simulink model "comparacao"  (R2018a)
settings: Solver=ode45  StartTime=0.0  StopTime=1  RelTol=1e-5  EnableMultiTasking=on
undefined symbols (not defined in the file): KIm, Km, KPm, Pm, Ts
libraries: simulink x10
settings Model: Creator=dwbertol  LastModifiedBy=bruno
settings DataIOCC: LimitDataPoints=on  SaveFormat=Array  SignalLoggingSaveFormat=ModelDataLogs
settings OptimizationCC: ExpressionDepthLimit=2147483647  LifeSpan=inf
settings DebuggingCC: UnderspecifiedInitializationDetection=Classic  MergeDetectMultiDrivingBlocksExec=none  SolverPrmCheckMsg=warning  FcnCallInpInsideContextMsg=warning  StateNameClashWarn=warning  SFUnexpectedBacktrackingDiag=warning  SFNoUnconditionalDefaultTransitionDiag=warning  SFExecutionAtInitializationDiag=none
settings HardwareCC: ProdBitPerPointer=32  ProdBitPerSizeT=32  ProdBitPerPtrDiffT=32  ProdLargestAtomicFloat=None  ProdIntDivRoundTo=Undefined  ProdEndianess=Unspecified  ProdWordSize=32  ProdHWDeviceType=32-bit Generic
settings ModelReferenceCC: PropagateSignalLabelsOutOfModel=off
settings CodeAppCC: StateflowObjectComments=on
settings GRTTargetCC: TargetLangStandard=C89/C90 (ANSI)  GeneratePreprocessorConditionals=Disable all  CombineOutputUpdateFcns=off  GRTInterface=on
settings ConfigComp: CovMetricSettings=dw  CovHtmlReporting=on  CovSaveCumulativeToWorkspaceVar=on  CovSaveSingleToWorkspaceVar=on  CovExternalEMLEnable=off

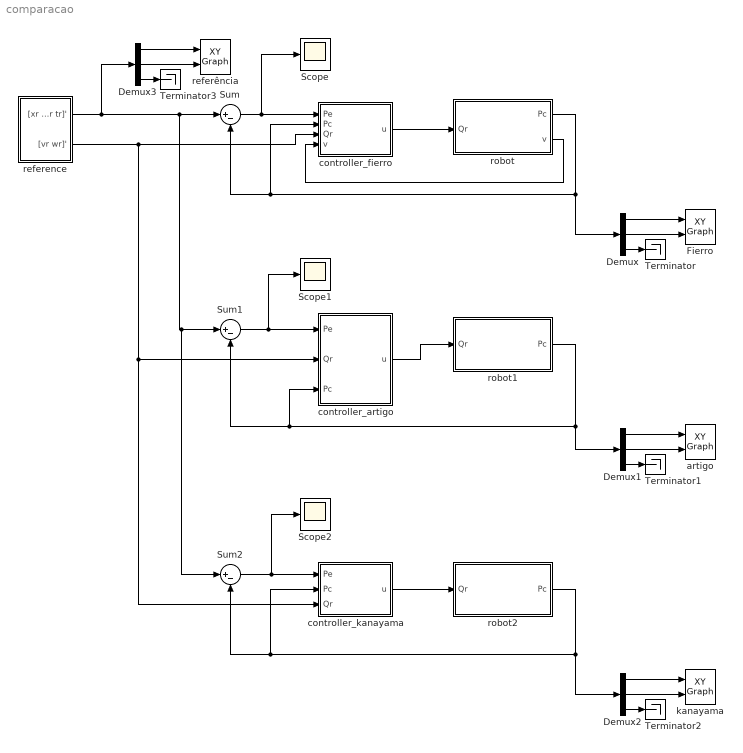
== system comparacao ==
  Demux{,1..3} (4 alike) : Demux  Outputs=3
  Fierro : simulink/Sinks/XY Graph  xmin=-0.1  xmax=1.1  ymin=-0.1  ymax=0.1  st=Ts
  Scope : Scope
  Scope1 : Scope
  Scope2 : Scope
  Sum : Sum  Inputs=|+-  AccumDataTypeStr=double
  Sum1 : Sum  Inputs=|+-  AccumDataTypeStr=double
  Sum2 : Sum  Inputs=|+-  AccumDataTypeStr=double
  Terminator{,1..3} (4 alike) : Terminator
  artigo : simulink/Sinks/XY Graph  xmin=-0.1  xmax=1.1  ymin=-0.1  ymax=0.1  st=Ts
  controller_artigo : Subsystem  mask{k1=60, k2=1000}
  controller_fierro : Subsystem  mask{kx=80, ky=2000, kt=160, k4=400}
  controller_kanayama : Subsystem  mask{kx=80, ky=2000, kt=160}
  kanayama : simulink/Sinks/XY Graph  xmin=-0.1  xmax=1.1  ymin=-0.1  ymax=0.1  st=Ts
  reference : Subsystem  mask{vr=1, wr=0, ini=[0 0.04 0], Ts=Ts}
  referência : simulink/Sinks/XY Graph  xmin=-0.1  xmax=1.1  ymin=-0.1  ymax=0.1  st=Ts
  robot : Subsystem  mask{ini=[0 0 0]'}
  robot1 : Subsystem  mask{ini=[0 0 0]'}
  robot2 : Subsystem  mask{ini=[0 0 0]'}
  wires:
  controller_fierro/1(u) -> robot/1(Qr)
  Demux/3 -> Terminator/1
  Demux/2 -> Fierro/2
  Demux/1 -> Fierro/1
  reference/1("[xr yr tr]' ") -> Demux3/1, Sum2/1, Sum1/1, Sum/1
  Sum/1 -> Scope/1, controller_fierro/1(Pe)
  reference/2("[vr wr]'") -> controller_artigo/2(Qr), controller_kanayama/3(Qr), controller_fierro/3(Qr)
  robot/1(Pc) -> Demux/1, Sum/2, controller_fierro/2(Pc)
  robot/2(v) -> controller_fierro/4(v)
  Demux1/1 -> artigo/1
  Sum1/1 -> Scope1/1, controller_artigo/1(Pe)
  robot1/1(Pc) -> Demux1/1, controller_artigo/3(Pc), Sum1/2
  Demux1/3 -> Terminator1/1
  controller_artigo/1(u) -> robot1/1(Qr)
  Demux1/2 -> artigo/2
  Demux2/1 -> kanayama/1
  Sum2/1 -> Scope2/1, controller_kanayama/1(Pe)
  Demux2/2 -> kanayama/2
  robot2/1(Pc) -> Demux2/1, Sum2/2, controller_kanayama/2(Pc)
  controller_kanayama/1(u) -> robot2/1(Qr)
  Demux2/3 -> Terminator2/1
  Demux3/1 -> referência/1
  Demux3/3 -> Terminator3/1
  Demux3/2 -> referência/2

== system comparacao/controller_artigo ==
  Pe : Inport
  Qr : Inport  Port=2
  Pc : Inport  Port=3
  Constant : Constant  Value=k1
  Constant1 : Constant  Value=k2
  controller : MATLAB Function  TreatAsAtomicUnit=on
  u : Outport
  wires:
  Qr/1 -> controller/2(Qr)
  Pe/1 -> controller/1(Pe)
  controller/1(u) -> u/1
  Constant/1 -> controller/4(k1)
  Constant1/1 -> controller/5(k2)
  Pc/1 -> controller/3(Pc)

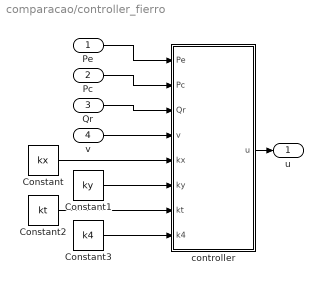
== system comparacao/controller_fierro ==
  Pe : Inport
  Pc : Inport  Port=2
  Qr : Inport  Port=3
  v : Inport  Port=4
  Constant : Constant  Value=kx
  Constant1 : Constant  Value=ky
  Constant2 : Constant  Value=kt
  Constant3 : Constant  Value=k4
  controller : MATLAB Function  TreatAsAtomicUnit=on
  u : Outport
  wires:
  controller/1(u) -> u/1
  Pe/1 -> controller/1(Pe)
  Pc/1 -> controller/2(Pc)
  Qr/1 -> controller/3(Qr)
  v/1 -> controller/4(v)
  Constant/1 -> controller/5(kx)
  Constant1/1 -> controller/6(ky)
  Constant2/1 -> controller/7(kt)
  Constant3/1 -> controller/8(k4)

== system comparacao/controller_kanayama ==
  Pe : Inport
  Pc : Inport  Port=2
  Qr : Inport  Port=3
  controller : MATLAB Function  TreatAsAtomicUnit=on
  u : Outport
  wires:
  Qr/1 -> controller/3(Qr)
  Pc/1 -> controller/2(Pc)
  Pe/1 -> controller/1(Pe)
  controller/1(u) -> u/1

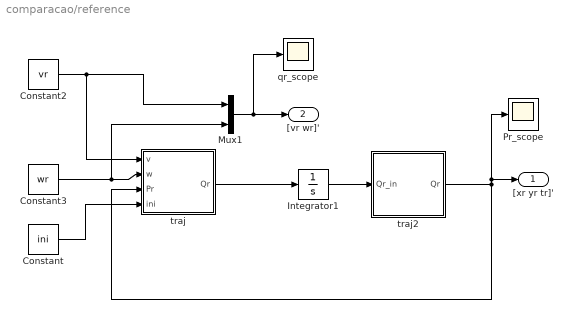
== system comparacao/reference ==
  Constant : Constant  Value=ini
  Constant2 : Constant  Value=vr  VectorParams1D=off
  Constant3 : Constant  Value=wr  VectorParams1D=off
  Integrator1 : Integrator  InitialCondition=ini
  Mux1 : Mux  Inputs=2
  Pr_scope : Scope
  qr_scope : Scope
  traj : MATLAB Function  TreatAsAtomicUnit=on
  traj2 : MATLAB Function  TreatAsAtomicUnit=on
  "[xr yr tr]' " : Outport
  "[vr wr]'" : Outport  Port=2
  wires:
  Integrator1/1 -> traj2/1(Qr_in)
  Constant3/1 -> Mux1/2, traj/2(w)
  Constant2/1 -> traj/1(v), Mux1/1
  Mux1/1 -> "[vr wr]'"/1, qr_scope/1
  traj/1(Qr) -> Integrator1/1
  Constant/1 -> traj/4(ini)
  traj2/1(Qr) -> Pr_scope/1, "[xr yr tr]' "/1, traj/3(Pr)

== system comparacao/robot ==
  Qr : Inport
  Controle velocidades : Subsystem
  Demux2 : Demux  Outputs=[2 1]
  Integrator1 : Integrator  InitialCondition=ini
  J : MATLAB Function  TreatAsAtomicUnit=on
  Terminator : Terminator
  Pc : Outport
  v : Outport  Port=2
  wires:
  J/1(P_ponto) -> Integrator1/1
  Integrator1/1 -> Demux2/1, Pc/1
  Demux2/1 -> Terminator/1
  Qr/1 -> Controle velocidades/1(Qr)
  Controle velocidades/1(Qc) -> v/1, J/1(Qc)
  Demux2/2 -> J/2(teta)

== system comparacao/robot1 ==
  Qr : Inport
  Controle velocidades : Subsystem
  Demux2 : Demux  Outputs=[2 1]
  Integrator1 : Integrator  InitialCondition=ini
  J : MATLAB Function  TreatAsAtomicUnit=on
  Terminator : Terminator
  Pc : Outport
  wires:
  J/1(P_ponto) -> Integrator1/1
  Integrator1/1 -> Demux2/1, Pc/1
  Demux2/1 -> Terminator/1
  Qr/1 -> Controle velocidades/1(Qr)
  Controle velocidades/1(Qc) -> J/1(Qc)
  Demux2/2 -> J/2(teta)

== system comparacao/robot2 ==
  Qr : Inport
  Controle velocidades : Subsystem
  Demux2 : Demux  Outputs=[2 1]
  Integrator1 : Integrator  InitialCondition=ini
  J : MATLAB Function  TreatAsAtomicUnit=on
  Terminator : Terminator
  vel : Scope
  Pc : Outport
  wires:
  J/1(P_ponto) -> vel/1, Integrator1/1
  Integrator1/1 -> Demux2/1, Pc/1
  Demux2/1 -> Terminator/1
  Qr/1 -> Controle velocidades/1(Qr)
  Controle velocidades/1(Qc) -> J/1(Qc)
  Demux2/2 -> J/2(teta)

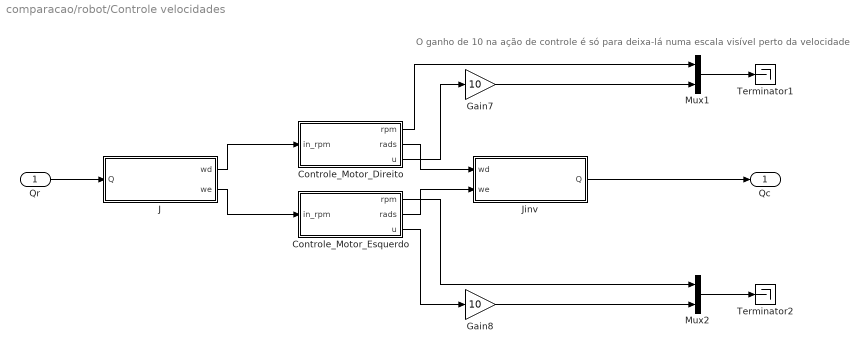
== system comparacao/robot/Controle velocidades ==
  note: O ganho de 10 na ação de controle é só para deixa-lá numa escala visível perto da velocidade
  Qr : Inport
  Controle_Motor_Direito : Subsystem
  Controle_Motor_Esquerdo : Subsystem
  Gain7 : Gain  Gain=10
  Gain8 : Gain  Gain=10
  J : MATLAB Function  TreatAsAtomicUnit=on
  Jinv : MATLAB Function  TreatAsAtomicUnit=on
  Mux1 : Mux  Inputs=2
  Mux2 : Mux  Inputs=2
  Terminator1 : Terminator
  Terminator2 : Terminator
  Qc : Outport
  wires:
  Gain7/1 -> Mux1/2
  Mux2/1 -> Terminator2/1
  Mux1/1 -> Terminator1/1
  Gain8/1 -> Mux2/2
  Controle_Motor_Direito/3(u) -> Gain7/1
  Controle_Motor_Direito/1(rpm) -> Mux1/1
  Controle_Motor_Esquerdo/3(u) -> Gain8/1
  Controle_Motor_Esquerdo/1(rpm) -> Mux2/1
  Qr/1 -> J/1(Q)
  J/1(wd) -> Controle_Motor_Direito/1(in_rpm)
  J/2(we) -> Controle_Motor_Esquerdo/1(in_rpm)
  Controle_Motor_Direito/2(rads) -> Jinv/1(wd)
  Controle_Motor_Esquerdo/2(rads) -> Jinv/2(we)
  Jinv/1(Q) -> Qc/1

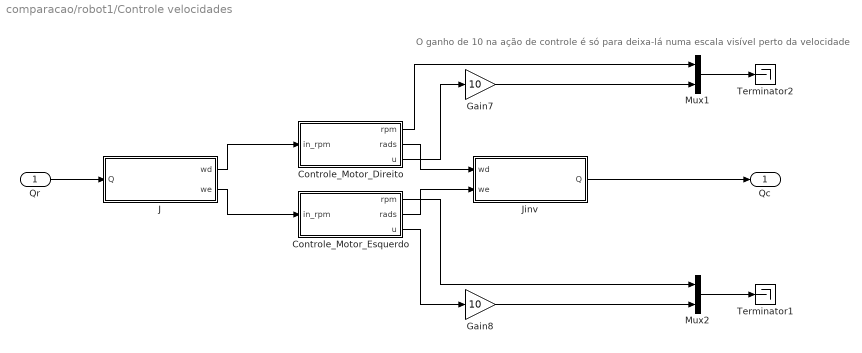
== system comparacao/robot1/Controle velocidades ==
  note: O ganho de 10 na ação de controle é só para deixa-lá numa escala visível perto da velocidade
  Qr : Inport
  Controle_Motor_Direito : Subsystem
  Controle_Motor_Esquerdo : Subsystem
  Gain7 : Gain  Gain=10
  Gain8 : Gain  Gain=10
  J : MATLAB Function  TreatAsAtomicUnit=on
  Jinv : MATLAB Function  TreatAsAtomicUnit=on
  Mux1 : Mux  Inputs=2
  Mux2 : Mux  Inputs=2
  Terminator1 : Terminator
  Terminator2 : Terminator
  Qc : Outport
  wires:
  Gain7/1 -> Mux1/2
  Mux2/1 -> Terminator1/1
  Mux1/1 -> Terminator2/1
  Gain8/1 -> Mux2/2
  Controle_Motor_Direito/3(u) -> Gain7/1
  Controle_Motor_Direito/1(rpm) -> Mux1/1
  Controle_Motor_Esquerdo/3(u) -> Gain8/1
  Controle_Motor_Esquerdo/1(rpm) -> Mux2/1
  Qr/1 -> J/1(Q)
  J/1(wd) -> Controle_Motor_Direito/1(in_rpm)
  J/2(we) -> Controle_Motor_Esquerdo/1(in_rpm)
  Controle_Motor_Direito/2(rads) -> Jinv/1(wd)
  Controle_Motor_Esquerdo/2(rads) -> Jinv/2(we)
  Jinv/1(Q) -> Qc/1

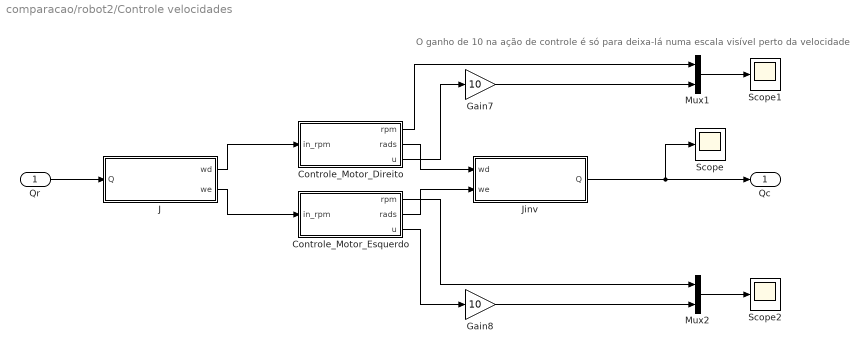
== system comparacao/robot2/Controle velocidades ==
  note: O ganho de 10 na ação de controle é só para deixa-lá numa escala visível perto da velocidade
  Qr : Inport
  Controle_Motor_Direito : Subsystem
  Controle_Motor_Esquerdo : Subsystem
  Gain7 : Gain  Gain=10
  Gain8 : Gain  Gain=10
  J : MATLAB Function  TreatAsAtomicUnit=on
  Jinv : MATLAB Function  TreatAsAtomicUnit=on
  Mux1 : Mux  Inputs=2
  Mux2 : Mux  Inputs=2
  Scope : Scope
  Scope1 : Scope
  Scope2 : Scope
  Qc : Outport
  wires:
  Gain7/1 -> Mux1/2
  Mux2/1 -> Scope2/1
  Mux1/1 -> Scope1/1
  Gain8/1 -> Mux2/2
  Controle_Motor_Direito/3(u) -> Gain7/1
  Controle_Motor_Direito/1(rpm) -> Mux1/1
  Controle_Motor_Esquerdo/3(u) -> Gain8/1
  Controle_Motor_Esquerdo/1(rpm) -> Mux2/1
  Qr/1 -> J/1(Q)
  J/1(wd) -> Controle_Motor_Direito/1(in_rpm)
  J/2(we) -> Controle_Motor_Esquerdo/1(in_rpm)
  Controle_Motor_Direito/2(rads) -> Jinv/1(wd)
  Controle_Motor_Esquerdo/2(rads) -> Jinv/2(we)
  Jinv/1(Q) -> Scope/1, Qc/1

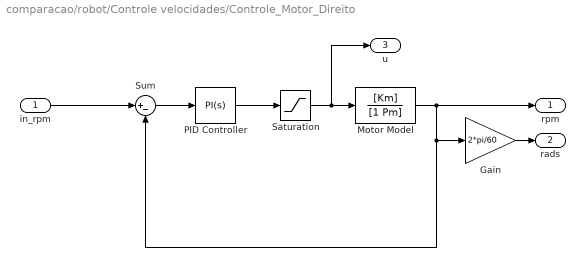
== system comparacao/robot/Controle velocidades/Controle_Motor_Direito ==
  in_rpm : Inport
  Gain : Gain  Gain=2*pi/60
  Motor Model : TransferFcn  Numerator=[Km]  Denominator=[1 Pm]
  PID Controller : simulink/Continuous/PID Controller  Controller=PI  TimeDomain=Continuous-time  SampleTime=-1  IntegratorMethod=Forward Euler  FilterMethod=Forward Euler  Form=Parallel  UseFilter=on  ControllerParametersSource=internal  P=KPm  I=KIm  D=0  N=0  InitialConditionSource=internal  InitialConditionForIntegrator=0  InitialConditionForFilter=0  ExternalReset=none  LimitOutput=off  UpperSaturationLimit=inf  LowerSaturationLimit=-inf  LinearizeAsGain=on  AntiWindupMode=none  Kb=1  TrackingMode=off  Kt=1  PParamMin=[]  PParamMax=[]  IParamMin=[]  IParamMax=[]  DParamMin=[]  DParamMax=[]  NParamMin=[]  NParamMax=[]  KbParamMin=[]  KbParamMax=[]  KtParamMin=[]  KtParamMax=[]  POutMin=[]  POutMax=[]  IOutMin=[]  IOutMax=[]  DOutMin=[]  DOutMax=[]  NOutMin=[]  NOutMax=[]  KbOutMin=[]  KbOutMax=[]  KtOutMin=[]  KtOutMax=[]  IntegratorOutMin=[]  IntegratorOutMax=[]  FilterOutMin=[]  FilterOutMax=[]  SumOutMin=[]  SumOutMax=[]  SumI1OutMin=[]  SumI1OutMax=[]  SumI2OutMin=[]  SumI2OutMax=[]  SumI3OutMin=[]  SumI3OutMax=[]  SumDOutMin=[]  SumDOutMax=[]  SaturationOutMin=[]  SaturationOutMax=[]  IntegratorContinuousStateAttributes=''  IntegratorStateMustResolveToSignalObject=off  IntegratorRTWStateStorageClass=Auto  FilterContinuousStateAttributes=''  FilterStateMustResolveToSignalObject=off  FilterRTWStateStorageClass=Auto  DifferentiatorICPrevScaledInput=0  DifferentiatorOutMin=[]  DifferentiatorOutMax=[]  FilterDiffOutCoefMin=[]  FilterDiffOutCoefMax=[]  SumDenOutMin=[]  SumDenOutMax=[]  SumNumOutMin=[]  SumNumOutMax=[]  ReciprocalOutMin=[]  ReciprocalOutMax=[]  DivideOutMin=[]  DivideOutMax=[]  TunerSelectOption=Transfer Function Based (PID Tuner App)
  Saturation : Saturate  UpperLimit=100  LowerLimit=-100
  Sum : Sum  Inputs=|+-
  rpm : Outport
  rads : Outport  Port=2
  u : Outport  Port=3
  wires:
  PID Controller/1 -> Saturation/1
  Motor Model/1 -> rpm/1, Gain/1, Sum/2
  Saturation/1 -> u/1, Motor Model/1
  Sum/1 -> PID Controller/1
  in_rpm/1 -> Sum/1
  Gain/1 -> rads/1

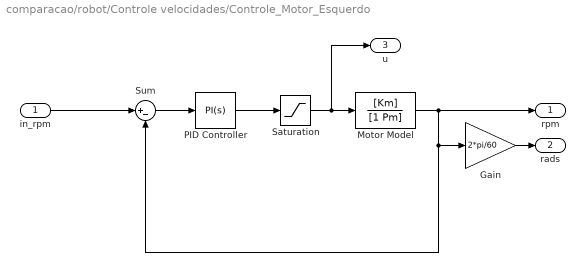
== system comparacao/robot/Controle velocidades/Controle_Motor_Esquerdo ==
  in_rpm : Inport
  Gain : Gain  Gain=2*pi/60
  Motor Model : TransferFcn  Numerator=[Km]  Denominator=[1 Pm]
  PID Controller : simulink/Continuous/PID Controller  Controller=PI  TimeDomain=Continuous-time  SampleTime=-1  IntegratorMethod=Forward Euler  FilterMethod=Forward Euler  Form=Parallel  UseFilter=on  ControllerParametersSource=internal  P=KPm  I=KIm  D=0  N=0  InitialConditionSource=internal  InitialConditionForIntegrator=0  InitialConditionForFilter=0  ExternalReset=none  LimitOutput=off  UpperSaturationLimit=inf  LowerSaturationLimit=-inf  LinearizeAsGain=on  AntiWindupMode=none  Kb=1  TrackingMode=off  Kt=1  PParamMin=[]  PParamMax=[]  IParamMin=[]  IParamMax=[]  DParamMin=[]  DParamMax=[]  NParamMin=[]  NParamMax=[]  KbParamMin=[]  KbParamMax=[]  KtParamMin=[]  KtParamMax=[]  POutMin=[]  POutMax=[]  IOutMin=[]  IOutMax=[]  DOutMin=[]  DOutMax=[]  NOutMin=[]  NOutMax=[]  KbOutMin=[]  KbOutMax=[]  KtOutMin=[]  KtOutMax=[]  IntegratorOutMin=[]  IntegratorOutMax=[]  FilterOutMin=[]  FilterOutMax=[]  SumOutMin=[]  SumOutMax=[]  SumI1OutMin=[]  SumI1OutMax=[]  SumI2OutMin=[]  SumI2OutMax=[]  SumI3OutMin=[]  SumI3OutMax=[]  SumDOutMin=[]  SumDOutMax=[]  SaturationOutMin=[]  SaturationOutMax=[]  IntegratorContinuousStateAttributes=''  IntegratorStateMustResolveToSignalObject=off  IntegratorRTWStateStorageClass=Auto  FilterContinuousStateAttributes=''  FilterStateMustResolveToSignalObject=off  FilterRTWStateStorageClass=Auto  DifferentiatorICPrevScaledInput=0  DifferentiatorOutMin=[]  DifferentiatorOutMax=[]  FilterDiffOutCoefMin=[]  FilterDiffOutCoefMax=[]  SumDenOutMin=[]  SumDenOutMax=[]  SumNumOutMin=[]  SumNumOutMax=[]  ReciprocalOutMin=[]  ReciprocalOutMax=[]  DivideOutMin=[]  DivideOutMax=[]  TunerSelectOption=Transfer Function Based (PID Tuner App)
  Saturation : Saturate  UpperLimit=100  LowerLimit=-100
  Sum : Sum  Inputs=|+-
  rpm : Outport
  rads : Outport  Port=2
  u : Outport  Port=3
  wires:
  PID Controller/1 -> Saturation/1
  Saturation/1 -> u/1, Motor Model/1
  Sum/1 -> PID Controller/1
  in_rpm/1 -> Sum/1
  Motor Model/1 -> rpm/1, Gain/1, Sum/2
  Gain/1 -> rads/1

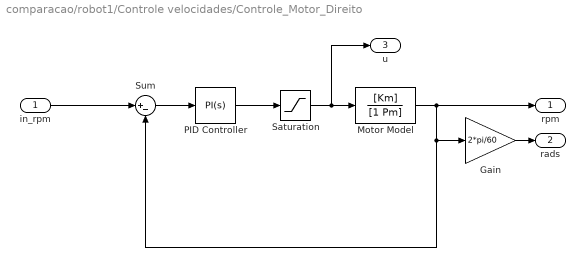
== system comparacao/robot1/Controle velocidades/Controle_Motor_Direito ==
  in_rpm : Inport
  Gain : Gain  Gain=2*pi/60
  Motor Model : TransferFcn  Numerator=[Km]  Denominator=[1 Pm]
  PID Controller : simulink/Continuous/PID Controller  Controller=PI  TimeDomain=Continuous-time  SampleTime=-1  IntegratorMethod=Forward Euler  FilterMethod=Forward Euler  Form=Parallel  UseFilter=on  ControllerParametersSource=internal  P=KPm  I=KIm  D=0  N=0  InitialConditionSource=internal  InitialConditionForIntegrator=0  InitialConditionForFilter=0  ExternalReset=none  LimitOutput=off  UpperSaturationLimit=inf  LowerSaturationLimit=-inf  LinearizeAsGain=on  AntiWindupMode=none  Kb=1  TrackingMode=off  Kt=1  PParamMin=[]  PParamMax=[]  IParamMin=[]  IParamMax=[]  DParamMin=[]  DParamMax=[]  NParamMin=[]  NParamMax=[]  KbParamMin=[]  KbParamMax=[]  KtParamMin=[]  KtParamMax=[]  POutMin=[]  POutMax=[]  IOutMin=[]  IOutMax=[]  DOutMin=[]  DOutMax=[]  NOutMin=[]  NOutMax=[]  KbOutMin=[]  KbOutMax=[]  KtOutMin=[]  KtOutMax=[]  IntegratorOutMin=[]  IntegratorOutMax=[]  FilterOutMin=[]  FilterOutMax=[]  SumOutMin=[]  SumOutMax=[]  SumI1OutMin=[]  SumI1OutMax=[]  SumI2OutMin=[]  SumI2OutMax=[]  SumI3OutMin=[]  SumI3OutMax=[]  SumDOutMin=[]  SumDOutMax=[]  SaturationOutMin=[]  SaturationOutMax=[]  IntegratorContinuousStateAttributes=''  IntegratorStateMustResolveToSignalObject=off  IntegratorRTWStateStorageClass=Auto  FilterContinuousStateAttributes=''  FilterStateMustResolveToSignalObject=off  FilterRTWStateStorageClass=Auto  DifferentiatorICPrevScaledInput=0  DifferentiatorOutMin=[]  DifferentiatorOutMax=[]  FilterDiffOutCoefMin=[]  FilterDiffOutCoefMax=[]  SumDenOutMin=[]  SumDenOutMax=[]  SumNumOutMin=[]  SumNumOutMax=[]  ReciprocalOutMin=[]  ReciprocalOutMax=[]  DivideOutMin=[]  DivideOutMax=[]  TunerSelectOption=Transfer Function Based (PID Tuner App)
  Saturation : Saturate  UpperLimit=100  LowerLimit=-100
  Sum : Sum  Inputs=|+-
  rpm : Outport
  rads : Outport  Port=2
  u : Outport  Port=3
  wires:
  PID Controller/1 -> Saturation/1
  Motor Model/1 -> rpm/1, Gain/1, Sum/2
  Saturation/1 -> u/1, Motor Model/1
  Sum/1 -> PID Controller/1
  in_rpm/1 -> Sum/1
  Gain/1 -> rads/1

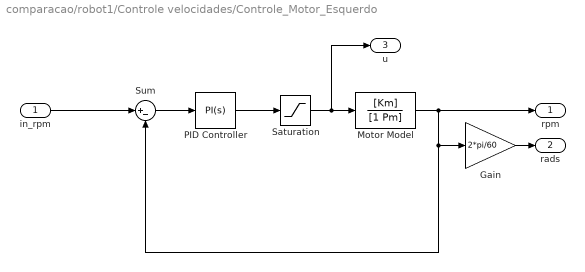
== system comparacao/robot1/Controle velocidades/Controle_Motor_Esquerdo ==
  in_rpm : Inport
  Gain : Gain  Gain=2*pi/60
  Motor Model : TransferFcn  Numerator=[Km]  Denominator=[1 Pm]
  PID Controller : simulink/Continuous/PID Controller  Controller=PI  TimeDomain=Continuous-time  SampleTime=-1  IntegratorMethod=Forward Euler  FilterMethod=Forward Euler  Form=Parallel  UseFilter=on  ControllerParametersSource=internal  P=KPm  I=KIm  D=0  N=0  InitialConditionSource=internal  InitialConditionForIntegrator=0  InitialConditionForFilter=0  ExternalReset=none  LimitOutput=off  UpperSaturationLimit=inf  LowerSaturationLimit=-inf  LinearizeAsGain=on  AntiWindupMode=none  Kb=1  TrackingMode=off  Kt=1  PParamMin=[]  PParamMax=[]  IParamMin=[]  IParamMax=[]  DParamMin=[]  DParamMax=[]  NParamMin=[]  NParamMax=[]  KbParamMin=[]  KbParamMax=[]  KtParamMin=[]  KtParamMax=[]  POutMin=[]  POutMax=[]  IOutMin=[]  IOutMax=[]  DOutMin=[]  DOutMax=[]  NOutMin=[]  NOutMax=[]  KbOutMin=[]  KbOutMax=[]  KtOutMin=[]  KtOutMax=[]  IntegratorOutMin=[]  IntegratorOutMax=[]  FilterOutMin=[]  FilterOutMax=[]  SumOutMin=[]  SumOutMax=[]  SumI1OutMin=[]  SumI1OutMax=[]  SumI2OutMin=[]  SumI2OutMax=[]  SumI3OutMin=[]  SumI3OutMax=[]  SumDOutMin=[]  SumDOutMax=[]  SaturationOutMin=[]  SaturationOutMax=[]  IntegratorContinuousStateAttributes=''  IntegratorStateMustResolveToSignalObject=off  IntegratorRTWStateStorageClass=Auto  FilterContinuousStateAttributes=''  FilterStateMustResolveToSignalObject=off  FilterRTWStateStorageClass=Auto  DifferentiatorICPrevScaledInput=0  DifferentiatorOutMin=[]  DifferentiatorOutMax=[]  FilterDiffOutCoefMin=[]  FilterDiffOutCoefMax=[]  SumDenOutMin=[]  SumDenOutMax=[]  SumNumOutMin=[]  SumNumOutMax=[]  ReciprocalOutMin=[]  ReciprocalOutMax=[]  DivideOutMin=[]  DivideOutMax=[]  TunerSelectOption=Transfer Function Based (PID Tuner App)
  Saturation : Saturate  UpperLimit=100  LowerLimit=-100
  Sum : Sum  Inputs=|+-
  rpm : Outport
  rads : Outport  Port=2
  u : Outport  Port=3
  wires:
  PID Controller/1 -> Saturation/1
  Saturation/1 -> u/1, Motor Model/1
  Sum/1 -> PID Controller/1
  in_rpm/1 -> Sum/1
  Motor Model/1 -> rpm/1, Gain/1, Sum/2
  Gain/1 -> rads/1

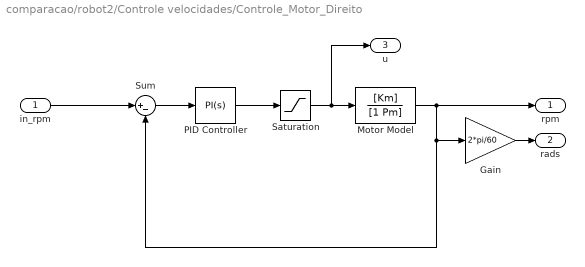
== system comparacao/robot2/Controle velocidades/Controle_Motor_Direito ==
  in_rpm : Inport
  Gain : Gain  Gain=2*pi/60
  Motor Model : TransferFcn  Numerator=[Km]  Denominator=[1 Pm]
  PID Controller : simulink/Continuous/PID Controller  Controller=PI  TimeDomain=Continuous-time  SampleTime=-1  IntegratorMethod=Forward Euler  FilterMethod=Forward Euler  Form=Parallel  UseFilter=on  ControllerParametersSource=internal  P=KPm  I=KIm  D=0  N=0  InitialConditionSource=internal  InitialConditionForIntegrator=0  InitialConditionForFilter=0  ExternalReset=none  LimitOutput=off  UpperSaturationLimit=inf  LowerSaturationLimit=-inf  LinearizeAsGain=on  AntiWindupMode=none  Kb=1  TrackingMode=off  Kt=1  PParamMin=[]  PParamMax=[]  IParamMin=[]  IParamMax=[]  DParamMin=[]  DParamMax=[]  NParamMin=[]  NParamMax=[]  KbParamMin=[]  KbParamMax=[]  KtParamMin=[]  KtParamMax=[]  POutMin=[]  POutMax=[]  IOutMin=[]  IOutMax=[]  DOutMin=[]  DOutMax=[]  NOutMin=[]  NOutMax=[]  KbOutMin=[]  KbOutMax=[]  KtOutMin=[]  KtOutMax=[]  IntegratorOutMin=[]  IntegratorOutMax=[]  FilterOutMin=[]  FilterOutMax=[]  SumOutMin=[]  SumOutMax=[]  SumI1OutMin=[]  SumI1OutMax=[]  SumI2OutMin=[]  SumI2OutMax=[]  SumI3OutMin=[]  SumI3OutMax=[]  SumDOutMin=[]  SumDOutMax=[]  SaturationOutMin=[]  SaturationOutMax=[]  IntegratorContinuousStateAttributes=''  IntegratorStateMustResolveToSignalObject=off  IntegratorRTWStateStorageClass=Auto  FilterContinuousStateAttributes=''  FilterStateMustResolveToSignalObject=off  FilterRTWStateStorageClass=Auto  DifferentiatorICPrevScaledInput=0  DifferentiatorOutMin=[]  DifferentiatorOutMax=[]  FilterDiffOutCoefMin=[]  FilterDiffOutCoefMax=[]  SumDenOutMin=[]  SumDenOutMax=[]  SumNumOutMin=[]  SumNumOutMax=[]  ReciprocalOutMin=[]  ReciprocalOutMax=[]  DivideOutMin=[]  DivideOutMax=[]  TunerSelectOption=Transfer Function Based (PID Tuner App)
  Saturation : Saturate  UpperLimit=100  LowerLimit=-100
  Sum : Sum  Inputs=|+-
  rpm : Outport
  rads : Outport  Port=2
  u : Outport  Port=3
  wires:
  PID Controller/1 -> Saturation/1
  Motor Model/1 -> rpm/1, Gain/1, Sum/2
  Saturation/1 -> u/1, Motor Model/1
  Sum/1 -> PID Controller/1
  in_rpm/1 -> Sum/1
  Gain/1 -> rads/1

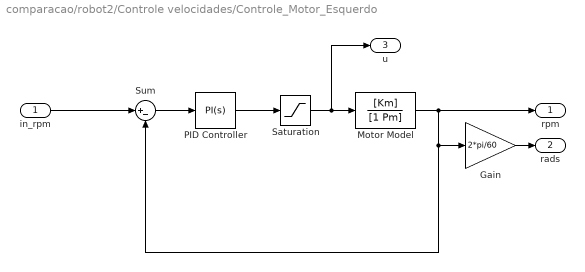
== system comparacao/robot2/Controle velocidades/Controle_Motor_Esquerdo ==
  in_rpm : Inport
  Gain : Gain  Gain=2*pi/60
  Motor Model : TransferFcn  Numerator=[Km]  Denominator=[1 Pm]
  PID Controller : simulink/Continuous/PID Controller  Controller=PI  TimeDomain=Continuous-time  SampleTime=-1  IntegratorMethod=Forward Euler  FilterMethod=Forward Euler  Form=Parallel  UseFilter=on  ControllerParametersSource=internal  P=KPm  I=KIm  D=0  N=0  InitialConditionSource=internal  InitialConditionForIntegrator=0  InitialConditionForFilter=0  ExternalReset=none  LimitOutput=off  UpperSaturationLimit=inf  LowerSaturationLimit=-inf  LinearizeAsGain=on  AntiWindupMode=none  Kb=1  TrackingMode=off  Kt=1  PParamMin=[]  PParamMax=[]  IParamMin=[]  IParamMax=[]  DParamMin=[]  DParamMax=[]  NParamMin=[]  NParamMax=[]  KbParamMin=[]  KbParamMax=[]  KtParamMin=[]  KtParamMax=[]  POutMin=[]  POutMax=[]  IOutMin=[]  IOutMax=[]  DOutMin=[]  DOutMax=[]  NOutMin=[]  NOutMax=[]  KbOutMin=[]  KbOutMax=[]  KtOutMin=[]  KtOutMax=[]  IntegratorOutMin=[]  IntegratorOutMax=[]  FilterOutMin=[]  FilterOutMax=[]  SumOutMin=[]  SumOutMax=[]  SumI1OutMin=[]  SumI1OutMax=[]  SumI2OutMin=[]  SumI2OutMax=[]  SumI3OutMin=[]  SumI3OutMax=[]  SumDOutMin=[]  SumDOutMax=[]  SaturationOutMin=[]  SaturationOutMax=[]  IntegratorContinuousStateAttributes=''  IntegratorStateMustResolveToSignalObject=off  IntegratorRTWStateStorageClass=Auto  FilterContinuousStateAttributes=''  FilterStateMustResolveToSignalObject=off  FilterRTWStateStorageClass=Auto  DifferentiatorICPrevScaledInput=0  DifferentiatorOutMin=[]  DifferentiatorOutMax=[]  FilterDiffOutCoefMin=[]  FilterDiffOutCoefMax=[]  SumDenOutMin=[]  SumDenOutMax=[]  SumNumOutMin=[]  SumNumOutMax=[]  ReciprocalOutMin=[]  ReciprocalOutMax=[]  DivideOutMin=[]  DivideOutMax=[]  TunerSelectOption=Transfer Function Based (PID Tuner App)
  Saturation : Saturate  UpperLimit=100  LowerLimit=-100
  Sum : Sum  Inputs=|+-
  rpm : Outport
  rads : Outport  Port=2
  u : Outport  Port=3
  wires:
  PID Controller/1 -> Saturation/1
  Saturation/1 -> u/1, Motor Model/1
  Sum/1 -> PID Controller/1
  in_rpm/1 -> Sum/1
  Motor Model/1 -> rpm/1, Gain/1, Sum/2
  Gain/1 -> rads/1

== matlab function comparacao/controller_artigo/controller ==
  data: Pe input; Qr input; Pc input; k1 input; u output; k2 input
function u = fcn(Pe,Qr,Pc,k1,k2)

Pe = -Pe;
% Pe = -[cos(Pc(3)) sin(Pc(3)) 0; -sin(Pc(3)) cos(Pc(3)) 0; 0 0 1]*Pe;

if Pe(3) ~= 0
    w = -k1*Pe(3) - k2*Pe(2)*Qr(1)*sin(Pe(3))/Pe(3);
else
    w = - k2*Pe(2)*Qr(1);
end

u = [Qr(1); w];
 
end

== matlab function comparacao/robot/Controle velocidades/J ==
  data: Q input; wd output; we output
function [wd, we] = fcn(Q)
% Dados do robô
r = 16e-3;      % Raio da roda
a = 69e-3;      % Distância do centro do robô até o centro das rodas

w_mot_rpm = (60/(2*pi))*[1/r a/r; 1/r -a/r]*Q;   % o 60/(2pi) é pra converter p/ rpm
wd = w_mot_rpm(1);
we = w_mot_rpm(2);

== matlab function comparacao/robot/Controle velocidades/Jinv ==
  data: wd input; Q output; we input
function Q = fcn(wd, we)
% Dados do robô
r = 16e-3;      % Raio da roda
a = 69e-3;      % Distância do centro do robô até o centro das rodas

Q = (r/2)*[1 1; 1/a -1/a]*[wd; we];

== matlab function comparacao/controller_fierro/controller ==
  data: Pe input size=3; Pc input size=3; Qr input size=2; v input size=2; u output size=2; kx input; ky input; kt input; k4 input
function u = fcn(Pe,Pc,Qr,v,kx,ky,kt,k4)

e = [cos(Pc(3)) sin(Pc(3)) 0; -sin(Pc(3)) cos(Pc(3)) 0; 0 0 1]*Pe;
%  Pe(1) = 0;  %essa linha é um caso a parte (para o seguidor de linha)

Qc = [Qr(1)*cos(e(3))+kx*e(1);Qr(2)+ky*Qr(1)*e(2)+kt*Qr(1)*sin(e(3))];
 
ep = [v(2)*e(2)-v(1)+Qr(1)*cos(e(3));-v(2)*e(1)+Qr(1)*sin(e(3));Qr(2)-v(2)];
Qcp = [kx 0 -Qr(1)*sin(e(3)); 0 ky*Qr(1) kt*Qr(1)*cos(e(3))]*ep;
 
u = k4*(Qc-v) + Qcp;

% vc = Qr(1)*cos(e(3))+kx*e(1);
% wc = Qr(2)+ky*Qr(1)*e(2)+kt*Qr(1)*sin(e(3));
% 
% xep = v(2)*e(2)-v(1)+Qr(1)*cos(e(3));
% yep = -v(2)*e(1)+Qr(1)*sin(e(3));
% tetaep = Qr(2)-v(2);
% 
% vcp = kx*xep - tetaep*Qr(1)*sin(e(3));
% wcp = ky*Qr(1)*yep + kt*Qr(1)*cos(e(3))*tetaep;
% 
% u = [k4*(vc-v(1))+vcp; k4*(wc-v(2))+wcp];
 
end

== matlab function comparacao/robot/J ==
  data: Qc input size=2; P_ponto output size=3; teta input size=1
function P_ponto = fcn(Qc, teta)

P_ponto = [Qc(1)*cos(teta); Qc(1)*sin(teta); Qc(2)]; %[Vx, Vy, Vteta];

== matlab function comparacao/controller_kanayama/controller ==
  data: Pe input; Pc input; Qr input; u output; kx parameter; ky parameter; kt parameter
function u = fcn(Pe,Pc,Qr,kx,ky,kt)

 Pe = [cos(Pc(3)) sin(Pc(3)) 0; -sin(Pc(3)) cos(Pc(3)) 0; 0 0 1]*Pe;
%  Pe(1) = 0;  %essa linha é um caso a parte (para o seguidor de linha)
 u = [Qr(1)*cos(Pe(3))+kx*Pe(1) Qr(2)+Qr(1)*(ky*Pe(2)+kt*sin(Pe(3)))]';
 
end

== matlab function comparacao/reference/traj ==
  data: v input; w input; Pr input; Qr output; ini input
function Qr = fcn(v, w, Pr, ini)

 Qr = [cos(Pr(3)) 0; sin(Pr(3)) 0; 0 1]*[v; w];

 
end

== matlab function comparacao/robot1/Controle velocidades/J ==
  data: Q input; wd output; we output
function [wd, we] = fcn(Q)
% Dados do robô
r = 16e-3;      % Raio da roda
a = 69e-3;      % Distância do centro do robô até o centro das rodas

w_mot_rpm = (60/(2*pi))*[1/r a/r; 1/r -a/r]*Q;   % o 60/(2pi) é pra converter p/ rpm
wd = w_mot_rpm(1);
we = w_mot_rpm(2);

== matlab function comparacao/robot1/Controle velocidades/Jinv ==
  data: wd input; Q output; we input
function Q = fcn(wd, we)
% Dados do robô
r = 16e-3;      % Raio da roda
a = 69e-3;      % Distância do centro do robô até o centro das rodas

Q = (r/2)*[1 1; 1/a -1/a]*[wd; we];

== matlab function comparacao/robot1/J ==
  data: Qc input; P_ponto output; teta input
function P_ponto = fcn(Qc, teta)

P_ponto = [Qc(1)*cos(teta); Qc(1)*sin(teta); Qc(2)]; %[Vx, Vy, Vteta];

== matlab function comparacao/reference/traj2 ==
  data: Qr_in input; Qr output
function Qr = fcn(Qr_in)

 Qr = Qr_in;
 Qr(2) = sin(4*pi*Qr(1))/20;

 
end

== matlab function comparacao/robot2/Controle velocidades/J ==
  data: Q input; wd output; we output
function [wd, we] = fcn(Q)
% Dados do robô
r = 16e-3;      % Raio da roda
a = 69e-3;      % Distância do centro do robô até o centro das rodas

w_mot_rpm = (60/(2*pi))*[1/r a/r; 1/r -a/r]*Q;   % o 60/(2pi) é pra converter p/ rpm
wd = w_mot_rpm(1);
we = w_mot_rpm(2);

== matlab function comparacao/robot2/Controle velocidades/Jinv ==
  data: wd input; Q output; we input
function Q = fcn(wd, we)
% Dados do robô
r = 16e-3;      % Raio da roda
a = 69e-3;      % Distância do centro do robô até o centro das rodas

Q = (r/2)*[1 1; 1/a -1/a]*[wd; we];

== matlab function comparacao/robot2/J ==
  data: Qc input; P_ponto output; teta input
function P_ponto = fcn(Qc, teta)

P_ponto = [Qc(1)*cos(teta); Qc(1)*sin(teta); Qc(2)]; %[Vx, Vy, Vteta];
